simulink model "SS3"  (R2020a)
settings: Solver=VariableStepAuto  StartTime=0.0  StopTime=10.0  RelTol=1e-3
settings Model: Creator=Asus  LastModifiedBy=Asus

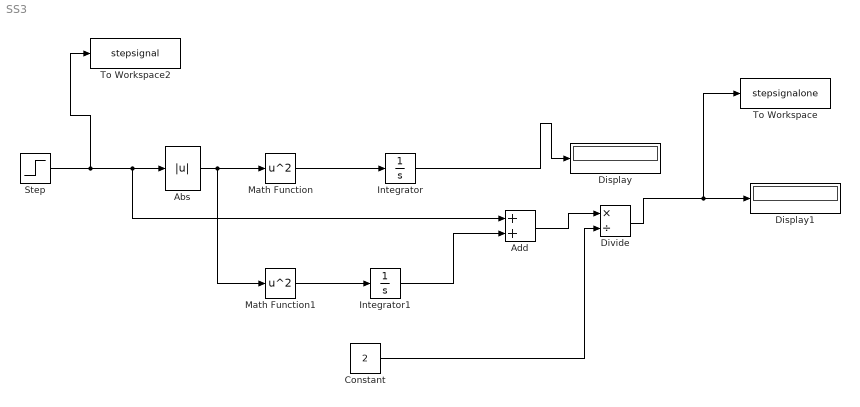
== system SS3 ==
  Abs : Abs
  Add : Sum
  Constant : Constant  Value=2
  Display : Display
  Display1 : Display
  Divide : Product  Inputs=*/
  Integrator : Integrator  LimitOutput=on
  Integrator1 : Integrator  LimitOutput=on
  Math Function : Math  Operator=square  SaturateOnIntegerOverflow=on
  Math Function1 : Math  Operator=square  SaturateOnIntegerOverflow=on
  Step : Step  SampleTime=0
  To Workspace : ToWorkspace  VariableName=stepsignalone  SaveFormat=Timeseries  SampleTime=-1
  To Workspace2 : ToWorkspace  VariableName=stepsignal  SaveFormat=Timeseries  SampleTime=-1
  wires:
  Constant/1 -> Divide/2
  Step/1 -> To Workspace2/1, Add/1, Abs/1
  Abs/1 -> Math Function1/1, Math Function/1
  Math Function/1 -> Integrator/1
  Integrator1/1 -> Add/2
  Divide/1 -> To Workspace/1, Display1/1
  Math Function1/1 -> Integrator1/1
  Integrator/1 -> Display/1
  Add/1 -> Divide/1
